simulink model "Simplified_UAV_Task3"  (R2024b)
settings: Solver=VariableStepAuto  StartTime=0  StopTime=3000  FixedStep=1e-4  RelTol=1e-5  AbsTol=1e-5
values from neighbouring files (symbols this model uses):
  adaptiveActivation = 1    [Simplified_UAV_Task3_main.m]    (also in newUAV_Task3_main.m)
  B_p = 1/UAV.m    [Simplified_UAV_Task3_main.m]    (also in newUAV_Task3_main.m)
  Gamma_a = 1*[1 1 1 1]'    [Simplified_UAV_Task3_main.m]    (also in newUAV_Task3_main.m = 2*[1 1 1 1]')
  gravityInAdaptiveController = 1    [Simplified_UAV_Task3_main.m]    (also in newUAV_Task3_main.m)
  L = 10    [Simplified_UAV_Task3_main.m]    (also in newUAV_Task3_main.m)
  lambda = 0.89    [Simplified_UAV_Task3_main.m]    (also in newUAV_Task3_main.m)
  lambda_0 = 1    [Simplified_UAV_Task3_main.m]    (also in newUAV_Task3_main.m)
  p_0 = [0; 0; 0]    [Simplified_UAV_Task3_main.m]    (also in newUAV_Task3_main.m)
  PO = 1    [Simplified_UAV_Task3_main.m]    (also in newUAV_Task3_main.m)
  scenario = 2    [Simplified_UAV_Task3_main.m]    (also in newUAV_Task3_main.m)
  theta_0 = [0.07;0.07;0.1]    [Simplified_UAV_Task3_main.m]    (also in newUAV_Task3_main.m)
  vb_0 = [0; 0; 0]    [Simplified_UAV_Task3_main.m]    (also in newUAV_Task3_main.m)
undefined symbols (not defined in the file or in its folder): ctrl, epsilon_PO, g, Gamma_a_scalar, par, projection_operator, targetParams, theta_M, UAV, v_0
libraries: matrix_library x12, slpidlib x12, spsRMSLib x1, uavutilslib x1
(part 1 of 3)
settings Model: Creator=justs  LastModifiedBy=giuseppe
settings SolverCC: ZeroCrossAlgorithm=Adaptive
settings DataIOCC: SaveFormat=StructureWithTime
settings OptimizationCC: BlockReduction=off  BufferReuse=off  ReuseModelBlockBuffer=off
settings DebuggingCC: AlgebraicLoopMsg=none
settings ModelReferenceCC: EnableRefExpFcnMdlSchedulingChecks=on
settings RTWCC: GPUComputeCapability=3.5

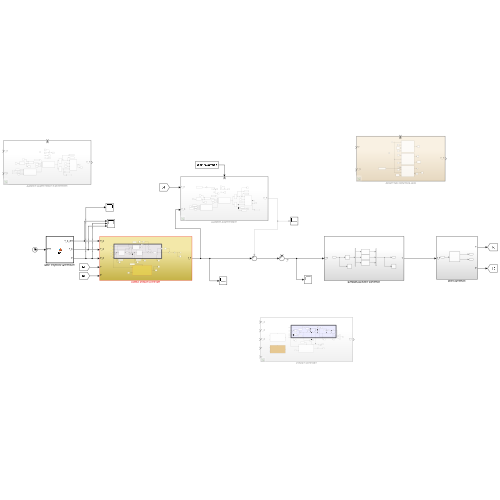
[thumbnail: Simulink's stored preview of the top-level diagram]
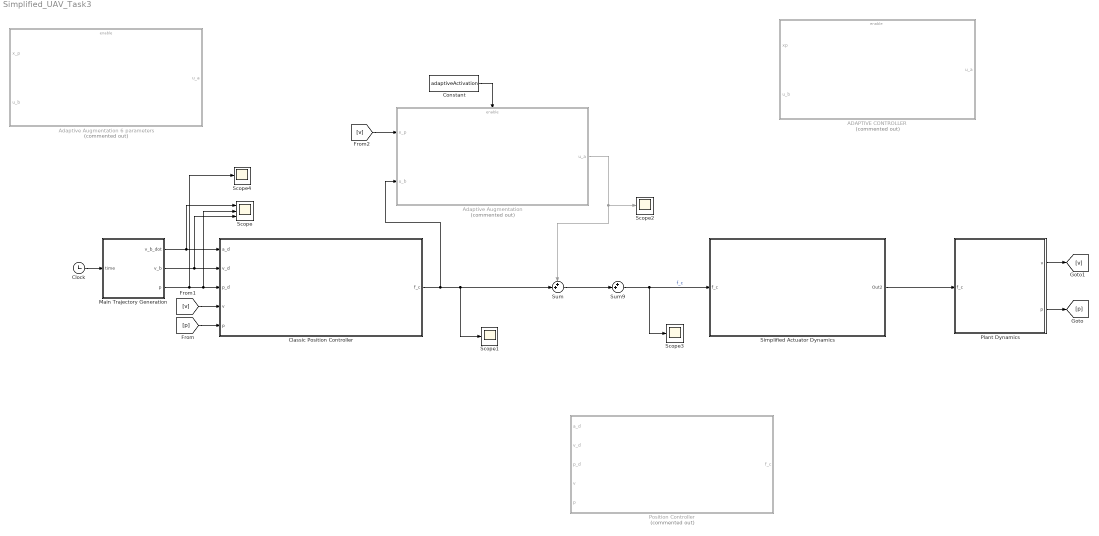
== system Simplified_UAV_Task3 ==
  ADAPTIVE CONTROLLER : Subsystem  Commented=on
  Adaptive Augmentation : Subsystem  Commented=on
  Adaptive Augmentation 6 parameters : Subsystem  Commented=on
  Classic Position Controller : Subsystem
  Clock : Clock
  Constant : Constant  Value=adaptiveActivation
  Main Trajectory Generation : MATLAB Function  TreatAsAtomicUnit=on
  Plant Dynamics : Subsystem
  Position Controller : Subsystem  Commented=on
  Scope : Scope  NumInputPorts=3
  Scope{1..4} (4 alike) : Scope
  Simplified Actuator Dynamics : Subsystem
  Sum : Sum  Inputs=++|
  Sum9 : Sum  Inputs=++|
  wires:
  Clock/1 -> Main Trajectory Generation/1(time)
  Simplified Actuator Dynamics/1(Out2) -> Plant Dynamics/1(f_c)
  Main Trajectory Generation/1(v_b_dot) -> Classic Position Controller/1(a_d), Scope/1
  Main Trajectory Generation/3(p) -> Scope4/1, Classic Position Controller/3(p_d), Scope/2
  Plant Dynamics/2(p) -> [p]
  [p] -> Classic Position Controller/5(p)
  Plant Dynamics/1(v) -> [v]
  [v] -> Classic Position Controller/4(v)
  Main Trajectory Generation/2(v_b) -> Classic Position Controller/2(v_d), Scope/3
  Classic Position Controller/1(f_c) -> Adaptive Augmentation/2(u_b), Scope1/1, Sum/2
  [v] -> Adaptive Augmentation/1(x_p)
  Adaptive Augmentation/1(u_a) -> Scope2/1, Sum/1
  Constant/1 -> Adaptive Augmentation/Enable
  Sum/1 -> Sum9/2
  Sum9/1 -> Scope3/1, Simplified Actuator Dynamics/1(f_c)  "f_c"

== system Simplified_UAV_Task3/ADAPTIVE CONTROLLER ==
  xp : Inport
  u_b : Inport  Port=2
  Enable : EnablePort
  Constant2 : Constant  Value=UAV.m*g*e3
  Scope : Scope
  Subsystem : Subsystem
  Subsystem1 : Subsystem
  Subsystem2 : Subsystem
  Sum : Sum  Inputs=|++
  u_a : Outport
  wires:
  Subsystem/1(xp_hat) -> [xp_hat]
  [thetap_hat] -> Subsystem1/4(thetap_hat)
  [thetap_hat] -> Subsystem/3(thetap_hat)
  xp/1 -> Subsystem1/3(xp), Subsystem2/2(xp), Subsystem/1(xp)
  [xp_hat] -> Subsystem2/3(xp_hat)
  [lambda] -> Subsystem/2(lambda)
  [u] -> Subsystem2/1(u)
  [u] -> Subsystem/4(u)
  Subsystem1/2(u) -> Scope/1, [u]
  [lambda] -> Subsystem1/2(lambda)
  Subsystem1/1(u_a) -> u_a/1
  Subsystem2/1(lambda) -> [lambda]
  Subsystem2/2(thetap_hat) -> [thetap_hat]
  Constant2/1 -> Sum/2
  u_b/1 -> Sum/1
  Sum/1 -> Subsystem1/1(u_b)

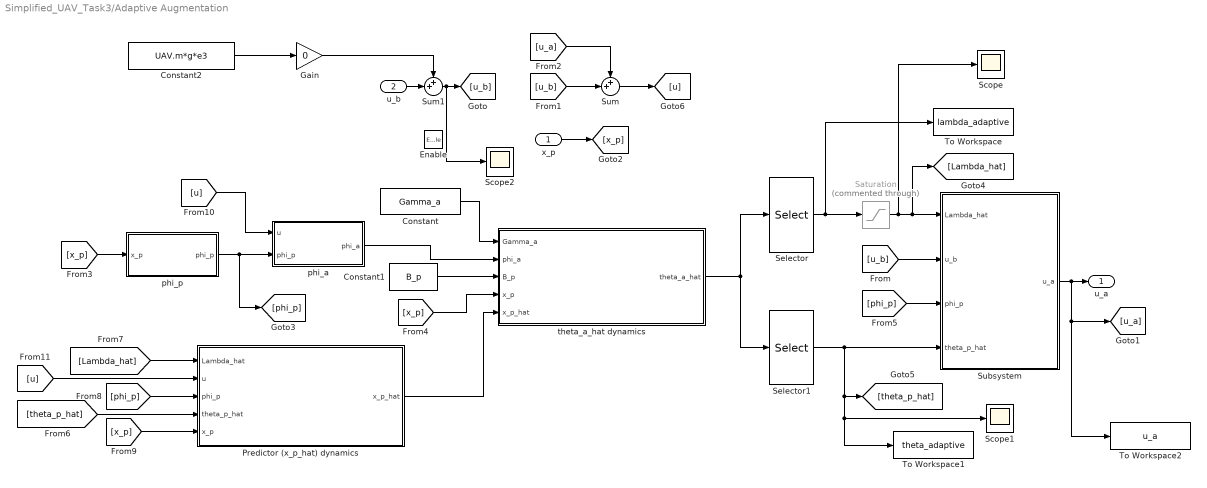
== system Simplified_UAV_Task3/Adaptive Augmentation ==
  x_p : Inport
  u_b : Inport  Port=2
  Enable : EnablePort
  Constant : Constant  Value=Gamma_a
  Constant1 : Constant  Value=B_p
  Constant2 : Constant  Value=UAV.m*g*e3
  Gain : Gain  Gain=0
  Predictor (x_p_hat) dynamics : Subsystem
  Saturation : Saturate  Commented=through  UpperLimit=1.5  LowerLimit=0.5
  Scope : Scope
  Scope1 : Scope
  Scope2 : Scope
  Selector : Selector  InputPortWidth=4  IndexOptions=Index vector (dialog)  Indices=[1]  OutputSizes=1
  Selector1 : Selector  InputPortWidth=4  IndexOptions=Index vector (dialog)  Indices=[2 3 4]  OutputSizes=1
  Subsystem : Subsystem
  Sum : Sum  Inputs=++|
  Sum1 : Sum  Inputs=++|
  To Workspace : ToWorkspace  VariableName=lambda_adaptive  SaveFormat=Timeseries  SampleTime=-1
  To Workspace1 : ToWorkspace  VariableName=theta_adaptive  SaveFormat=Timeseries  SampleTime=-1
  To Workspace2 : ToWorkspace  VariableName=u_a  SaveFormat=Timeseries  SampleTime=-1
  phi_a : Subsystem
  phi_p : Subsystem
  theta_a_hat dynamics : Subsystem
  u_a : Outport
  wires:
  Subsystem/1(u_a) -> To Workspace2/1, [u_a], u_a/1
  Selector1/1 -> Scope1/1, To Workspace1/1, [theta_p_hat], Subsystem/4(theta_p_hat)
  theta_a_hat dynamics/1(theta_a_hat) -> Selector/1, Selector1/1
  Constant/1 -> theta_a_hat dynamics/1(Gamma_a)
  phi_p/1(phi_p) -> phi_a/2(phi_p), [phi_p]
  [u_b] -> Sum/2
  phi_a/1(phi_a) -> theta_a_hat dynamics/2(phi_a)
  [x_p] -> phi_p/1(x_p)
  [x_p] -> theta_a_hat dynamics/4(x_p)
  Constant1/1 -> theta_a_hat dynamics/3(B_p)
  [phi_p] -> Subsystem/3(phi_p)
  Predictor (x_p_hat) dynamics/1(x_p_hat) -> theta_a_hat dynamics/5(x_p_hat)
  [theta_p_hat] -> Predictor (x_p_hat) dynamics/4(theta_p_hat)
  [Lambda_hat] -> Predictor (x_p_hat) dynamics/1(Lambda_hat)
  [phi_p] -> Predictor (x_p_hat) dynamics/3(phi_p)
  [x_p] -> Predictor (x_p_hat) dynamics/5(x_p)
  Sum/1 -> [u]
  [u] -> Predictor (x_p_hat) dynamics/2(u)
  Selector/1 -> To Workspace/1, Saturation/1
  x_p/1 -> [x_p]
  [u_a] -> Sum/1
  [u] -> phi_a/1(u)
  Saturation/1 -> Scope/1, [Lambda_hat], Subsystem/1(Lambda_hat)
  u_b/1 -> Sum1/2
  Sum1/1 -> Scope2/1, [u_b]
  Constant2/1 -> Gain/1
  Gain/1 -> Sum1/1
  [u_b] -> Subsystem/2(u_b)

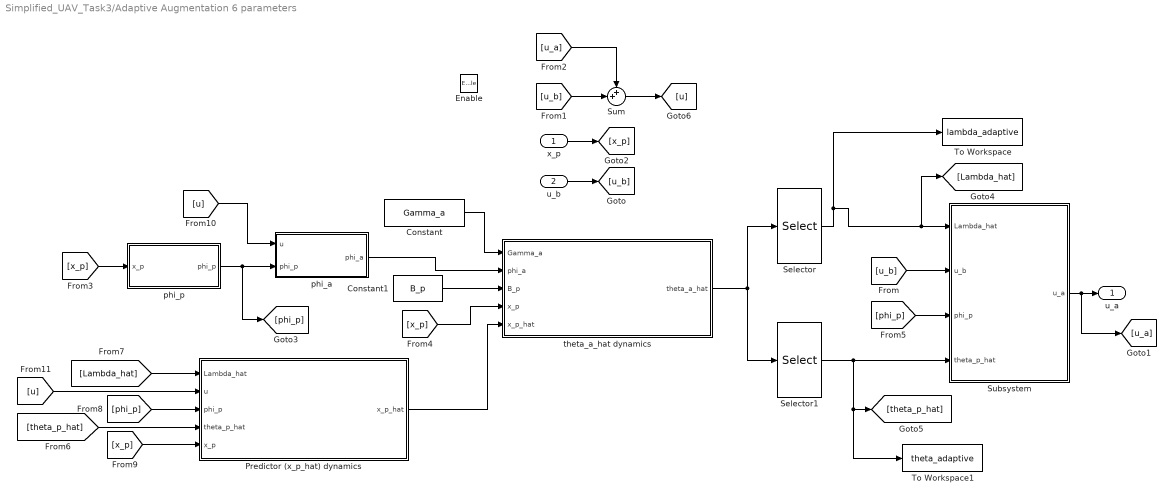
== system Simplified_UAV_Task3/Adaptive Augmentation 6 parameters ==
  x_p : Inport
  u_b : Inport  Port=2
  Enable : EnablePort
  Constant : Constant  Value=Gamma_a
  Constant1 : Constant  Value=B_p
  Predictor (x_p_hat) dynamics : Subsystem
  Selector : Selector  InputPortWidth=4  IndexOptions=Index vector (dialog)  Indices=[1]  OutputSizes=1
  Selector1 : Selector  InputPortWidth=4  IndexOptions=Index vector (dialog)  Indices=[2 3 4]  OutputSizes=1
  Subsystem : Subsystem
  Sum : Sum  Inputs=++|
  To Workspace : ToWorkspace  VariableName=lambda_adaptive  SaveFormat=Timeseries  SampleTime=-1
  To Workspace1 : ToWorkspace  VariableName=theta_adaptive  SaveFormat=Timeseries  SampleTime=-1
  phi_a : Subsystem
  phi_p : Subsystem
  theta_a_hat dynamics : Subsystem
  u_a : Outport
  wires:
  Subsystem/1(u_a) -> [u_a], u_a/1
  Selector1/1 -> To Workspace1/1, [theta_p_hat], Subsystem/4(theta_p_hat)
  theta_a_hat dynamics/1(theta_a_hat) -> Selector/1, Selector1/1
  Constant/1 -> theta_a_hat dynamics/1(Gamma_a)
  phi_p/1(phi_p) -> phi_a/2(phi_p), [phi_p]
  u_b/1 -> [u_b]
  [u_b] -> Subsystem/2(u_b)
  [u_b] -> Sum/2
  phi_a/1(phi_a) -> theta_a_hat dynamics/2(phi_a)
  [x_p] -> phi_p/1(x_p)
  [x_p] -> theta_a_hat dynamics/4(x_p)
  Constant1/1 -> theta_a_hat dynamics/3(B_p)
  [phi_p] -> Subsystem/3(phi_p)
  Predictor (x_p_hat) dynamics/1(x_p_hat) -> theta_a_hat dynamics/5(x_p_hat)
  [theta_p_hat] -> Predictor (x_p_hat) dynamics/4(theta_p_hat)
  [Lambda_hat] -> Predictor (x_p_hat) dynamics/1(Lambda_hat)
  [phi_p] -> Predictor (x_p_hat) dynamics/3(phi_p)
  [x_p] -> Predictor (x_p_hat) dynamics/5(x_p)
  Sum/1 -> [u]
  [u] -> Predictor (x_p_hat) dynamics/2(u)
  Selector/1 -> [Lambda_hat], Subsystem/1(Lambda_hat), To Workspace/1
  x_p/1 -> [x_p]
  [u_a] -> Sum/1
  [u] -> phi_a/1(u)

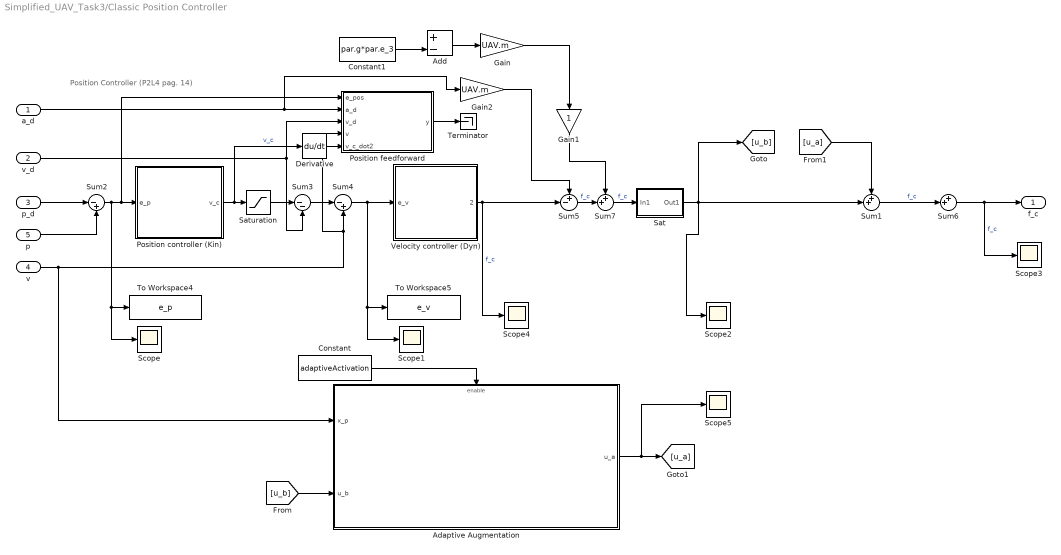
== system Simplified_UAV_Task3/Classic Position Controller ==
  note: Position Controller (P2L4 pag. 14)
  a_d : Inport
  v_d : Inport  Port=2
  p_d : Inport  Port=3
  v : Inport  Port=4
  p : Inport  Port=5
  Adaptive Augmentation : Subsystem
  Add : Sum  Inputs=+-
  Constant : Constant  Value=adaptiveActivation
  Constant1 : Constant  Value=par.g*par.e_3
  Derivative : Derivative
  Gain : Gain  Gain=UAV.m
  Gain1 : Gain
  Gain2 : Gain  Gain=UAV.m
  Position controller (Kin) : Subsystem
  Position feedforward : MATLAB Function  TreatAsAtomicUnit=on
  Sat : Subsystem
  Saturation : Saturate  UpperLimit=ctrl.vMax  LowerLimit=-ctrl.vMax
  Scope{,1..5} (6 alike) : Scope
  Sum1 : Sum  Inputs=++|
  Sum2 : Sum  Inputs=|-+
  Sum3 : Sum  Inputs=|--
  Sum4 : Sum  Inputs=|-+
  Sum5 : Sum  Inputs=+-|
  Sum6 : Sum  Inputs=++|
  Sum7 : Sum  Inputs=++|
  Terminator : Terminator
  To Workspace4 : ToWorkspace  VariableName=e_p  SaveFormat=Timeseries  SampleTime=-1
  To Workspace5 : ToWorkspace  VariableName=e_v  SaveFormat=Timeseries  SampleTime=-1
  Velocity controller (Dyn) : Subsystem
  f_c : Outport
  wires:
  p/1 -> Sum2/2
  a_d/1 -> Gain2/1, Position feedforward/2(a_d)
  Sum4/1 -> Scope1/1, To Workspace5/1, Velocity controller (Dyn)/1(e_v)
  v_d/1 -> Sum3/2, Position feedforward/3(v_d)
  p_d/1 -> Sum2/1
  Sum3/1 -> Sum4/1
  Sum2/1 -> Position feedforward/1(e_pos), Position controller (Kin)/1(e_p), Scope/1, To Workspace4/1
  Sum5/1 -> Sum7/2  "f_c"
  Position controller (Kin)/1(v_c) -> Derivative/1, Saturation/1  "v_c"
  Saturation/1 -> Sum3/1
  Velocity controller (Dyn)/1(2) -> Scope4/1, Sum5/2  "f_c"
  Derivative/1 -> Position feedforward/5(v_c_dot2)
  Position feedforward/1(y) -> Terminator/1
  Gain/1 -> Gain1/1
  Add/1 -> Gain/1
  Constant1/1 -> Add/2
  Sat/1(Out1) -> Scope2/1, [u_b], Sum1/2
  Gain1/1 -> Sum7/1
  Sum1/1 -> Sum6/2  "f_c"
  [u_b] -> Adaptive Augmentation/2(u_b)
  Adaptive Augmentation/1(u_a) -> Scope5/1, [u_a]
  [u_a] -> Sum1/1
  v/1 -> Adaptive Augmentation/1(x_p), Position feedforward/4(v), Sum4/2
  Constant/1 -> Adaptive Augmentation/Enable
  Sum6/1 -> Scope3/1, f_c/1  "f_c"
  Gain2/1 -> Sum5/1
  Sum7/1 -> Sat/1(In1)  "f_c"

== system Simplified_UAV_Task3/Plant Dynamics ==
  f_c : Inport
  Dynamics : Subsystem
  v : Outport
  p : Outport  Port=2
  wires:
  Dynamics/1(p) -> p/1
  Dynamics/2(v) -> v/1
  f_c/1 -> Dynamics/1(f_c)

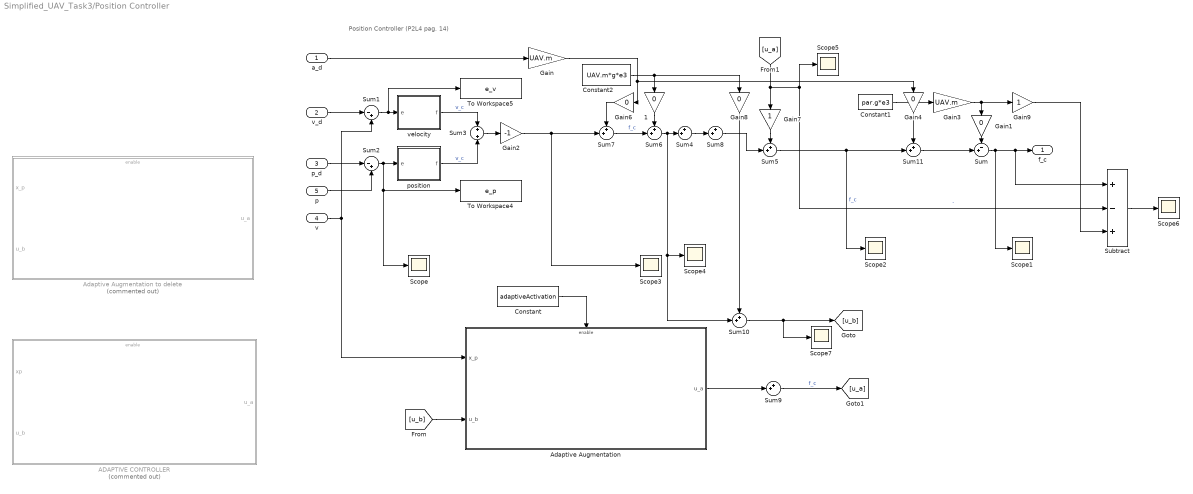
== system Simplified_UAV_Task3/Position Controller ==
  note: Position Controller (P2L4 pag. 14)
  a_d : Inport
  v_d : Inport  Port=2
  p_d : Inport  Port=3
  v : Inport  Port=4
  p : Inport  Port=5
  1 : Gain  Gain=0
  ADAPTIVE CONTROLLER : Subsystem  Commented=on
  Adaptive Augmentation : Subsystem
  Adaptive Augmentation to delete : Subsystem  Commented=on
  Constant : Constant  Value=adaptiveActivation
  "Constant1 " : Constant  Value=par.g*e3
  Constant2 : Constant  Value=UAV.m*g*e3
  Gain : Gain  Gain=UAV.m
  Gain{1,4,6,8} (4 alike) : Gain  Gain=0
  Gain2 : Gain  Gain=-1
  Gain3 : Gain  Gain=UAV.m
  Gain7 : Gain
  Gain9 : Gain
  Scope{,1..7} (8 alike) : Scope
  Subtract : Sum  Inputs=+-+
  Sum : Sum  Inputs=-+|
  Sum1 : Sum  Inputs=|-+
  Sum{4..11} (8 alike) : Sum  Inputs=++|
  Sum2 : Sum  Inputs=|-+
  Sum3 : Sum  Inputs=+|+
  To Workspace4 : ToWorkspace  VariableName=e_p  SaveFormat=Timeseries  SampleTime=-1
  To Workspace5 : ToWorkspace  VariableName=e_v  SaveFormat=Timeseries  SampleTime=-1
  position : Subsystem
  velocity : Subsystem
  f_c : Outport
  wires:
  p/1 -> Sum2/2
  v/1 -> Adaptive Augmentation/1(x_p), Sum1/2
  p_d/1 -> Sum2/1
  Sum2/1 -> position/1(e), Scope/1, To Workspace4/1
  Sum5/1 -> Sum11/2, Scope2/1  "f_c"
  Constant/1 -> Adaptive Augmentation/Enable
  [u_b] -> Adaptive Augmentation/2(u_b)
  [u_a] -> Subtract/2, Scope5/1, Gain7/1  "-"
  Gain/1 -> Gain6/1, Gain4/1
  a_d/1 -> Gain/1
  "Constant1 "/1 -> Gain3/1
  Sum/1 -> Scope1/1, Subtract/1, f_c/1
  v_d/1 -> Sum1/1
  Sum1/1 -> velocity/1(e), To Workspace5/1
  velocity/1(f) -> Sum3/1  "v_c"
  position/1(f) -> Sum3/2  "v_c"
  Sum3/1 -> Gain2/1
  Gain3/1 -> Gain9/1, Gain1/1
  Gain1/1 -> Sum/1
  Gain4/1 -> Sum11/1
  Gain2/1 -> Scope3/1, Sum7/2
  Constant2/1 -> Gain8/1, 1/1
  Sum7/1 -> Sum6/2  "f_c"
  Gain6/1 -> Sum7/1
  Gain7/1 -> Sum5/1
  Gain8/1 -> Sum10/1
  Sum4/1 -> Sum8/2
  Sum6/1 -> Sum10/2, Scope4/1, Sum4/2
  Subtract/1 -> Scope6/1
  Gain9/1 -> Subtract/3
  Adaptive Augmentation/1(u_a) -> Sum9/2
  Sum9/1 -> [u_a]  "f_c"
  Sum8/1 -> Sum5/2
  Sum10/1 -> Scope7/1, [u_b]
  1/1 -> Sum6/1
  Sum11/1 -> Sum/2

== system Simplified_UAV_Task3/Simplified Actuator Dynamics ==
  f_c : Inport
  Demux : Demux  Outputs=3
  Mux : Mux  Inputs=3
  Saturation : Saturate  UpperLimit=6  LowerLimit=-6
  Scope1 : Scope
  Scope2 : Scope
  Transfer Fcn : TransferFcn  Denominator=[1/70 1]
  Transfer Fcn1 : TransferFcn  Denominator=[1/10 1]
  Transfer Fcn2 : TransferFcn  Denominator=[1/10 1]
  Out2 : Outport
  wires:
  f_c/1 -> Saturation/1, Scope2/1
  Mux/1 -> Scope1/1, Out2/1
  Demux/1 -> Transfer Fcn2/1
  Demux/2 -> Transfer Fcn1/1
  Transfer Fcn/1 -> Mux/3
  Demux/3 -> Transfer Fcn/1
  Transfer Fcn1/1 -> Mux/2
  Transfer Fcn2/1 -> Mux/1
  Saturation/1 -> Demux/1

== system Simplified_UAV_Task3/ADAPTIVE CONTROLLER/Subsystem ==
  xp : Inport
  lambda : Inport  Port=2
  thetap_hat : Inport  Port=3
  u : Inport  Port=4
  Constant : Constant  Value=[0 0 g]'
  Create Diagonal Matrix : matrix_library/Create Diagonal Matrix
  Gain : Gain  Gain=B_p
  Gain1 : Gain  Gain=L
  Gain2 : Gain  Gain=-1
  Integrator : Integrator
  MATLAB Function1 : MATLAB Function  Commented=through  TreatAsAtomicUnit=on
  Matrix Multiply : Product  Multiplication=Matrix(*)
  Matrix Multiply1 : Product
  Scope : Scope
  Sum : Sum
  Sum1 : Sum  Inputs=+++
  Sum2 : Sum  Inputs=+-
  xp_hat : Outport
  wires:
  xp/1 -> Sum2/1, Create Diagonal Matrix/1
  thetap_hat/1 -> Matrix Multiply/2
  u/1 -> Matrix Multiply1/2
  MATLAB Function1/1(Lambda_hat) -> Matrix Multiply1/1
  lambda/1 -> MATLAB Function1/1(lambda)
  Sum/1 -> Gain/1
  Matrix Multiply1/1 -> Sum/1
  Matrix Multiply/1 -> Sum/2
  Gain/1 -> Sum1/2
  Constant/1 -> Sum1/1
  Integrator/1 -> xp_hat/1, Sum2/2
  Sum2/1 -> Scope/1, Gain1/1
  Gain1/1 -> Sum1/3
  Sum1/1 -> Integrator/1
  Create Diagonal Matrix/1 -> Gain2/1
  Gain2/1 -> Matrix Multiply/1

== system Simplified_UAV_Task3/ADAPTIVE CONTROLLER/Subsystem1 ==
  u_b : Inport
  lambda : Inport  Port=2
  xp : Inport  Port=3
  thetap_hat : Inport  Port=4
  Constant : Constant
  Create Diagonal Matrix : matrix_library/Create Diagonal Matrix
  Gain2 : Gain  Gain=-1
  MATLAB Function1 : MATLAB Function  TreatAsAtomicUnit=on
  Matrix Multiply : Product
  Matrix Multiply1 : Product  Multiplication=Matrix(*)
  Matrix Multiply2 : Product
  Sum : Sum  Inputs=+-
  Sum1 : Sum  Inputs=+-
  Sum2 : Sum
  u_a : Outport
  u : Outport  Port=2
  wires:
  lambda/1 -> MATLAB Function1/1(lambda)
  MATLAB Function1/1(Lambda_hat_inv) -> Matrix Multiply2/1, Sum/1
  Constant/1 -> Sum/2
  Sum/1 -> Matrix Multiply/1
  u_b/1 -> Sum2/2, Matrix Multiply/2
  Matrix Multiply/1 -> Sum1/1
  xp/1 -> Create Diagonal Matrix/1
  thetap_hat/1 -> Matrix Multiply1/2
  Sum1/1 -> Sum2/1, u_a/1
  Sum2/1 -> u/1
  Create Diagonal Matrix/1 -> Gain2/1
  Gain2/1 -> Matrix Multiply1/1
  Matrix Multiply1/1 -> Matrix Multiply2/2
  Matrix Multiply2/1 -> Sum1/2

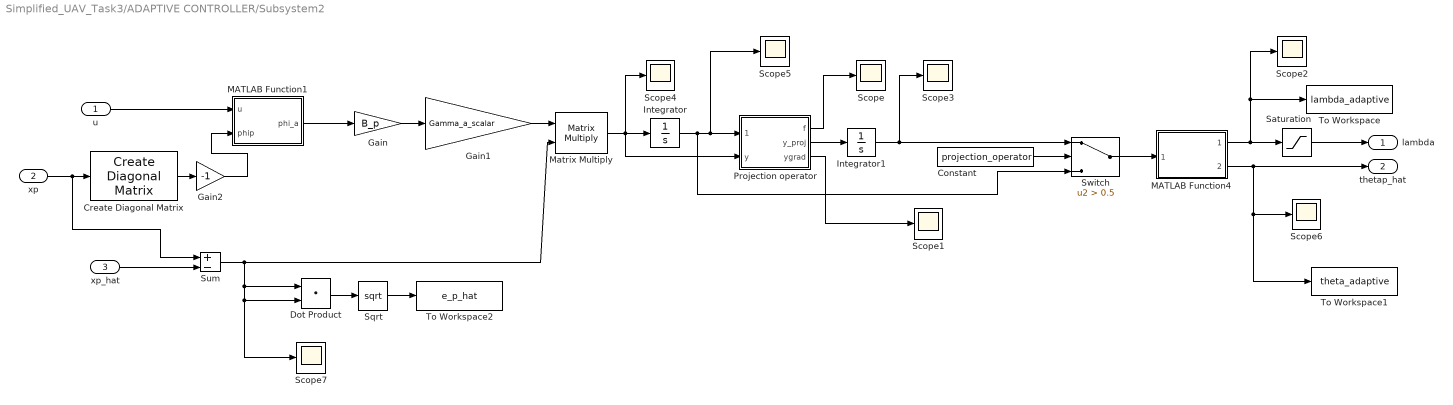
== system Simplified_UAV_Task3/ADAPTIVE CONTROLLER/Subsystem2 ==
  u : Inport
  xp : Inport  Port=2
  xp_hat : Inport  Port=3
  Constant : Constant  Value=projection_operator
  Create Diagonal Matrix : matrix_library/Create Diagonal Matrix
  Dot Product : DotProduct  OutDataTypeStr=Inherit: Inherit via internal rule
  Gain : Gain  Gain=B_p
  Gain1 : Gain  Gain=Gamma_a_scalar
  Gain2 : Gain  Gain=-1
  Integrator : Integrator  InitialCondition=[lambda_0; theta_0]
  Integrator1 : Integrator  InitialCondition=[1 0.07 0.07 0.1]'
  MATLAB Function1 : MATLAB Function  TreatAsAtomicUnit=on
  MATLAB Function4 : MATLAB Function  TreatAsAtomicUnit=on
  Matrix Multiply : Product  Multiplication=Matrix(*)
  Projection operator : MATLAB Function  TreatAsAtomicUnit=on
  Saturation : Saturate  UpperLimit=1.5  LowerLimit=0.5
  Scope{,1..7} (8 alike) : Scope
  Sqrt : Sqrt
  Sum : Sum  Inputs=+-
  Switch : Switch  Criteria=u2 > Threshold  Threshold=0.5  SaturateOnIntegerOverflow=off  InputSameDT=off
  To Workspace : ToWorkspace  VariableName=lambda_adaptive  SaveFormat=Timeseries  SampleTime=-1
  To Workspace1 : ToWorkspace  VariableName=theta_adaptive  SaveFormat=Timeseries  SampleTime=-1
  To Workspace2 : ToWorkspace  VariableName=e_p_hat  SaveFormat=Timeseries  SampleTime=-1
  lambda : Outport
  thetap_hat : Outport  Port=2
  wires:
  u/1 -> MATLAB Function1/1(u)
  xp_hat/1 -> Sum/2
  MATLAB Function1/1(phi_a) -> Gain/1
  Gain/1 -> Gain1/1
  Gain1/1 -> Matrix Multiply/1
  Matrix Multiply/1 -> Projection operator/2(y), Scope4/1, Integrator/1
  MATLAB Function4/1(lambda) -> To Workspace/1, Scope2/1, Saturation/1
  Integrator/1 -> Switch/3, Scope5/1, Projection operator/1(theta_a_hat)
  Projection operator/3(ygrad) -> Scope1/1
  Projection operator/1(f) -> Scope/1
  MATLAB Function4/2(thetap_hat) -> To Workspace1/1, Scope6/1, thetap_hat/1
  Integrator1/1 -> Switch/1, Scope3/1
  Projection operator/2(y_proj) -> Integrator1/1
  xp/1 -> Create Diagonal Matrix/1, Sum/1
  Switch/1 -> MATLAB Function4/1(theta_a)
  Constant/1 -> Switch/2
  Create Diagonal Matrix/1 -> Gain2/1
  Gain2/1 -> MATLAB Function1/2(phip)
  Sqrt/1 -> To Workspace2/1
  Sum/1 -> Scope7/1, Dot Product/2, Dot Product/1, Matrix Multiply/2
  Dot Product/1 -> Sqrt/1
  Saturation/1 -> lambda/1

== system Simplified_UAV_Task3/Adaptive Augmentation/Predictor (x_p_hat) dynamics ==
  Lambda_hat : Inport
  u : Inport  Port=2
  phi_p : Inport  Port=3
  theta_p_hat : Inport  Port=4
  x_p : Inport  Port=5
  Add : Sum
  Constant : Constant  Value=g*e3
  Gain : Gain  Gain=B_p  Multiplication=Matrix(K*u)
  Gain1 : Gain  Gain=L
  Gain2 : Gain  Gain=gravityInAdaptiveController
  Integrator : Integrator  InitialCondition=v_0
  Matrix Multiply : Product
  Matrix Multiply1 : Product  Multiplication=Matrix(*)
  Reshape : Reshape  OutputDimensionality=Column vector (2-D)
  Reshape1 : Reshape  OutputDimensionality=Column vector (2-D)
  Reshape2 : Reshape  OutputDimensionality=Column vector (2-D)
  Scope : Scope
  Sum : Sum  Inputs=+++
  Sum1 : Sum  Inputs=-+|
  Transpose : Math  Operator=transpose
  x_p_hat : Outport
  wires:
  Lambda_hat/1 -> Matrix Multiply/1
  Matrix Multiply/1 -> Add/1
  phi_p/1 -> Transpose/1
  theta_p_hat/1 -> Matrix Multiply1/2
  Matrix Multiply1/1 -> Add/2
  Add/1 -> Gain/1
  Gain/1 -> Reshape1/1
  Gain1/1 -> Reshape/1
  x_p/1 -> Sum1/2
  Sum1/1 -> Gain1/1
  Integrator/1 -> Scope/1, Sum1/1, x_p_hat/1
  Sum/1 -> Integrator/1
  Reshape/1 -> Sum/1
  Reshape1/1 -> Sum/2
  Reshape2/1 -> Sum/3
  Constant/1 -> Gain2/1
  Transpose/1 -> Matrix Multiply1/1
  Gain2/1 -> Reshape2/1
  u/1 -> Matrix Multiply/2

== system Simplified_UAV_Task3/Adaptive Augmentation/Subsystem ==
  Lambda_hat : Inport
  u_b : Inport  Port=2
  phi_p : Inport  Port=3
  theta_p_hat : Inport  Port=4
  Constant : Constant  Value=eye(3,3)
  Gain : Gain  Commented=through  Gain=-1
  Gain1 : Gain
  Inverse : MATLAB Function  TreatAsAtomicUnit=on
  Product : Product  Multiplication=Matrix(*)
  Product1 : Product  Inputs=3  Multiplication=Matrix(*)
  Subtract : Sum  Inputs=-+
  Subtract1 : Sum  Inputs=+-
  Transpose : Math  Operator=transpose
  u_a : Outport
  wires:
  Lambda_hat/1 -> Inverse/1(u)
  Inverse/1(y) -> Product1/1, Subtract/2
  Constant/1 -> Subtract/1
  Subtract/1 -> Product/1
  u_b/1 -> Product/2
  Product/1 -> Gain1/1
  Subtract1/1 -> u_a/1
  phi_p/1 -> Transpose/1
  Transpose/1 -> Gain/1
  theta_p_hat/1 -> Product1/3
  Product1/1 -> Subtract1/2
  Gain/1 -> Product1/2
  Gain1/1 -> Subtract1/1

== system Simplified_UAV_Task3/Adaptive Augmentation/phi_a ==
  u : Inport
  phi_p : Inport  Port=2
  Matrix Concatenate : Concatenate  Mode=Multidimensional array
  Scope : Scope
  Transpose : Math  Operator=transpose
  phi_a : Outport
  wires:
  Matrix Concatenate/1 -> Scope/1, phi_a/1
  u/1 -> Transpose/1
  phi_p/1 -> Matrix Concatenate/2
  Transpose/1 -> Matrix Concatenate/1

== system Simplified_UAV_Task3/Adaptive Augmentation/phi_p ==
  x_p : Inport
  Create Diagonal Matrix : matrix_library/Create Diagonal Matrix
  Gain : Gain  Gain=-1
  phi_p : Outport
  wires:
  x_p/1 -> Gain/1
  Gain/1 -> Create Diagonal Matrix/1
  Create Diagonal Matrix/1 -> phi_p/1

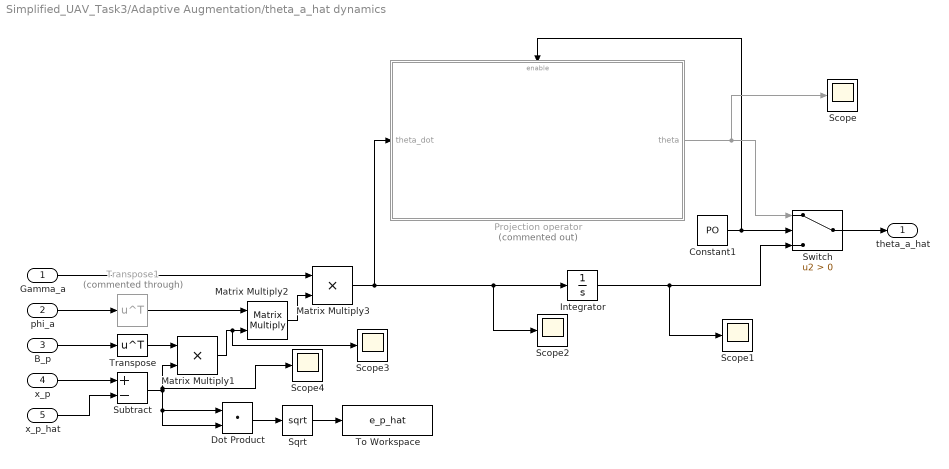
== system Simplified_UAV_Task3/Adaptive Augmentation/theta_a_hat dynamics ==
  Gamma_a : Inport
  phi_a : Inport  Port=2
  B_p : Inport  Port=3
  x_p : Inport  Port=4
  x_p_hat : Inport  Port=5
  Constant1 : Constant  Value=PO
  Dot Product : DotProduct  OutDataTypeStr=Inherit: Inherit via internal rule
  Integrator : Integrator  InitialCondition=[lambda_0; theta_0]
  Matrix Multiply1 : Product
  Matrix Multiply2 : Product  Multiplication=Matrix(*)
  Matrix Multiply3 : Product
  Projection operator : Subsystem  Commented=on
  Scope{,1..4} (5 alike) : Scope
  Sqrt : Sqrt
  Subtract : Sum  Inputs=+-
  Switch : Switch  Criteria=u2 > Threshold  SaturateOnIntegerOverflow=off  InputSameDT=off
  To Workspace : ToWorkspace  VariableName=e_p_hat  SaveFormat=Timeseries  SampleTime=-1
  Transpose : Math  Operator=transpose
  Transpose1 : Math  Commented=through  Operator=transpose
  theta_a_hat : Outport
  wires:
  x_p_hat/1 -> Subtract/2
  B_p/1 -> Transpose/1
  Subtract/1 -> Matrix Multiply1/2, Scope4/1, Dot Product/2, Dot Product/1
  Transpose/1 -> Matrix Multiply1/1
  phi_a/1 -> Transpose1/1
  Matrix Multiply1/1 -> Scope3/1, Matrix Multiply2/2
  Gamma_a/1 -> Matrix Multiply3/1
  Matrix Multiply2/1 -> Matrix Multiply3/2
  Matrix Multiply3/1 -> Projection operator/1(theta_dot), Scope2/1, Integrator/1
  x_p/1 -> Subtract/1
  Constant1/1 -> Switch/2, Projection operator/Enable
  Integrator/1 -> Scope1/1, Switch/3
  Switch/1 -> theta_a_hat/1
  Projection operator/1(theta) -> Scope/1, Switch/1
  Dot Product/1 -> Sqrt/1
  Sqrt/1 -> To Workspace/1
  Transpose1/1 -> Matrix Multiply2/1

== system Simplified_UAV_Task3/Adaptive Augmentation 6 parameters/Predictor (x_p_hat) dynamics ==
  Lambda_hat : Inport
  u : Inport  Port=2
  phi_p : Inport  Port=3
  theta_p_hat : Inport  Port=4
  x_p : Inport  Port=5
  Add : Sum
  Constant : Constant  Value=g*e3
  Gain : Gain  Gain=B_p  Multiplication=Matrix(K*u)
  Gain1 : Gain  Gain=L
  Integrator : Integrator  InitialCondition=v_0
  Matrix Multiply : Product  Multiplication=Matrix(*)
  Matrix Multiply1 : Product  Multiplication=Matrix(*)
  Reshape : Reshape  OutputDimensionality=Column vector (2-D)
  Reshape1 : Reshape  OutputDimensionality=Column vector (2-D)
  Reshape2 : Reshape  OutputDimensionality=Column vector (2-D)
  Sum : Sum  Inputs=+++
  Sum1 : Sum  Inputs=-+|
  Transpose : Math  Operator=transpose
  x_p_hat : Outport
  wires:
  Lambda_hat/1 -> Matrix Multiply/1
  u/1 -> Matrix Multiply/2
  Matrix Multiply/1 -> Add/1
  phi_p/1 -> Transpose/1
  theta_p_hat/1 -> Matrix Multiply1/2
  Matrix Multiply1/1 -> Add/2
  Transpose/1 -> Matrix Multiply1/1
  Add/1 -> Gain/1
  Gain/1 -> Reshape1/1
  Constant/1 -> Reshape2/1
  Gain1/1 -> Reshape/1
  x_p/1 -> Sum1/2
  Sum1/1 -> Gain1/1
  Integrator/1 -> Sum1/1, x_p_hat/1
  Sum/1 -> Integrator/1
  Reshape/1 -> Sum/1
  Reshape1/1 -> Sum/2
  Reshape2/1 -> Sum/3

== system Simplified_UAV_Task3/Adaptive Augmentation 6 parameters/Subsystem ==
  Lambda_hat : Inport
  u_b : Inport  Port=2
  phi_p : Inport  Port=3
  theta_p_hat : Inport  Port=4
  Constant : Constant  Value=eye(3,3)
  Inverse : MATLAB Function  TreatAsAtomicUnit=on
  Product : Product  Multiplication=Matrix(*)
  Product1 : Product  Multiplication=Matrix(*)
  Product2 : Product  Multiplication=Matrix(*)
  Subtract : Sum  Inputs=-+
  Subtract1 : Sum  Inputs=+-
  Transpose : Math  Operator=transpose
  u_a : Outport
  wires:
  Lambda_hat/1 -> Inverse/1(u)
  Inverse/1(y) -> Product1/1, Subtract/2
  Constant/1 -> Subtract/1
  Subtract/1 -> Product/1
  u_b/1 -> Product/2
  Product/1 -> Subtract1/1
  Subtract1/1 -> u_a/1
  phi_p/1 -> Transpose/1
  Transpose/1 -> Product2/1
  theta_p_hat/1 -> Product2/2
  Product2/1 -> Product1/2
  Product1/1 -> Subtract1/2

== system Simplified_UAV_Task3/Adaptive Augmentation 6 parameters/phi_a ==
  u : Inport
  phi_p : Inport  Port=2
  Create Diagonal Matrix : matrix_library/Create Diagonal Matrix
  Matrix Concatenate : Concatenate  Mode=Multidimensional array
  phi_a : Outport
  wires:
  phi_p/1 -> Matrix Concatenate/2
  u/1 -> Create Diagonal Matrix/1
  Matrix Concatenate/1 -> phi_a/1
  Create Diagonal Matrix/1 -> Matrix Concatenate/1

== system Simplified_UAV_Task3/Adaptive Augmentation 6 parameters/phi_p ==
  x_p : Inport
  Create Diagonal Matrix : matrix_library/Create Diagonal Matrix
  Gain : Gain  Gain=-1
  phi_p : Outport
  wires:
  x_p/1 -> Gain/1
  Gain/1 -> Create Diagonal Matrix/1
  Create Diagonal Matrix/1 -> phi_p/1

== system Simplified_UAV_Task3/Adaptive Augmentation 6 parameters/theta_a_hat dynamics ==
  Gamma_a : Inport
  phi_a : Inport  Port=2
  B_p : Inport  Port=3
  x_p : Inport  Port=4
  x_p_hat : Inport  Port=5
  Constant1 : Constant  Value=PO
  Integrator : Integrator  InitialCondition=[lambda_0; theta_0]
  Matrix Multiply1 : Product
  Matrix Multiply2 : Product  Multiplication=Matrix(*)
  Matrix Multiply3 : Product
  Projection operator : Subsystem  Commented=on
  Scope : Scope
  Subtract : Sum  Inputs=+-
  Switch : Switch  Criteria=u2 > Threshold  SaturateOnIntegerOverflow=off  InputSameDT=off
  Transpose : Math  Operator=transpose
  theta_a_hat : Outport
  wires:
  x_p_hat/1 -> Subtract/2
  B_p/1 -> Transpose/1
  Subtract/1 -> Matrix Multiply1/2
  Transpose/1 -> Matrix Multiply1/1
  phi_a/1 -> Matrix Multiply2/1
  Matrix Multiply1/1 -> Matrix Multiply2/2
  Gamma_a/1 -> Matrix Multiply3/1
  Matrix Multiply2/1 -> Matrix Multiply3/2
  Matrix Multiply3/1 -> Projection operator/1(theta_dot), Integrator/1
  x_p/1 -> Subtract/1
  Constant1/1 -> Switch/2, Projection operator/Enable
  Integrator/1 -> Switch/3
  Switch/1 -> theta_a_hat/1
  Projection operator/1(theta) -> Scope/1, Switch/1

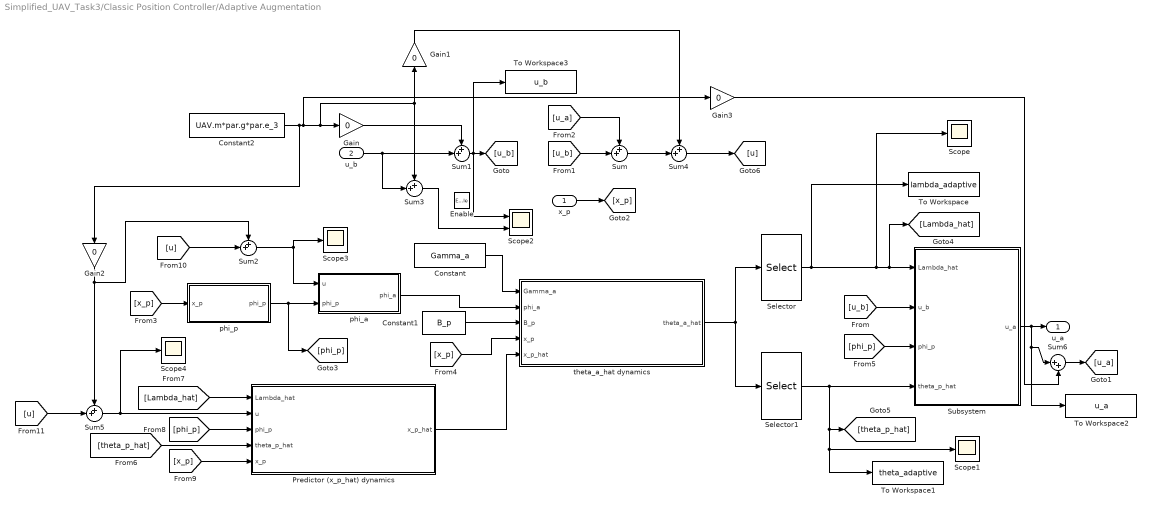
== system Simplified_UAV_Task3/Classic Position Controller/Adaptive Augmentation ==
  x_p : Inport
  u_b : Inport  Port=2
  Enable : EnablePort
  Constant : Constant  Value=Gamma_a
  Constant1 : Constant  Value=B_p
  Constant2 : Constant  Value=UAV.m*par.g*par.e_3
  Gain{,1..3} (4 alike) : Gain  Gain=0
  Predictor (x_p_hat) dynamics : Subsystem
  Scope{,1,3..4} (4 alike) : Scope
  Scope2 : Scope  NumInputPorts=2
  Selector : Selector  InputPortWidth=4  IndexOptions=Index vector (dialog)  Indices=[1]  OutputSizes=1
  Selector1 : Selector  InputPortWidth=4  IndexOptions=Index vector (dialog)  Indices=[2 3 4]  OutputSizes=1
  Subsystem : Subsystem
  Sum{,1..5} (6 alike) : Sum  Inputs=++|
  Sum6 : Sum  Inputs=|++
  To Workspace : ToWorkspace  VariableName=lambda_adaptive  SaveFormat=Timeseries  SampleTime=-1
  To Workspace1 : ToWorkspace  VariableName=theta_adaptive  SaveFormat=Timeseries  SampleTime=-1
  To Workspace2 : ToWorkspace  VariableName=u_a  SaveFormat=Timeseries  SampleTime=-1
  To Workspace3 : ToWorkspace  VariableName=u_b  SaveFormat=Timeseries  SampleTime=-1
  phi_a : Subsystem
  phi_p : Subsystem
  theta_a_hat dynamics : Subsystem
  u_a : Outport
  wires:
  Selector1/1 -> Scope1/1, To Workspace1/1, [theta_p_hat], Subsystem/4(theta_p_hat)
  theta_a_hat dynamics/1(theta_a_hat) -> Selector/1, Selector1/1
  Constant/1 -> theta_a_hat dynamics/1(Gamma_a)
  phi_p/1(phi_p) -> phi_a/2(phi_p), [phi_p]
  [u_b] -> Sum/2
  phi_a/1(phi_a) -> theta_a_hat dynamics/2(phi_a)
  [x_p] -> phi_p/1(x_p)
  [x_p] -> theta_a_hat dynamics/4(x_p)
  Constant1/1 -> theta_a_hat dynamics/3(B_p)
  [phi_p] -> Subsystem/3(phi_p)
  Predictor (x_p_hat) dynamics/1(x_p_hat) -> theta_a_hat dynamics/5(x_p_hat)
  [theta_p_hat] -> Predictor (x_p_hat) dynamics/4(theta_p_hat)
  [Lambda_hat] -> Predictor (x_p_hat) dynamics/1(Lambda_hat)
  [phi_p] -> Predictor (x_p_hat) dynamics/3(phi_p)
  [x_p] -> Predictor (x_p_hat) dynamics/5(x_p)
  x_p/1 -> [x_p]
  [u_a] -> Sum/1
  Selector/1 -> Scope/1, [Lambda_hat], Subsystem/1(Lambda_hat), To Workspace/1
  u_b/1 -> Sum3/2, Sum1/2
  Sum1/1 -> Scope2/1, To Workspace3/1, [u_b]
  [u_b] -> Subsystem/2(u_b)
  Subsystem/1(u_a) -> Sum6/1, To Workspace2/1, u_a/1
  Sum2/1 -> phi_a/1(u), Scope3/1
  [u] -> Sum2/2
  Gain/1 -> Sum1/1
  Sum3/1 -> Scope2/2
  Sum/1 -> Sum4/2
  Sum4/1 -> [u]
  Constant2/1 -> Gain2/1, Gain3/1, Gain1/1, Sum3/1, Gain/1
  Gain1/1 -> Sum4/1
  [u] -> Sum5/2
  Sum5/1 -> Scope4/1, Predictor (x_p_hat) dynamics/2(u)
  Gain2/1 -> Sum2/1, Sum5/1
  Sum6/1 -> [u_a]
  Gain3/1 -> Sum6/2

== system Simplified_UAV_Task3/Classic Position Controller/Position controller (Kin) ==
  e_p : Inport
  Constant : Constant  Value=scenario
  Demux : Demux  Outputs=3
  If : If  IfExpression=u1 == 2
  Mux : Mux  Inputs=3
  PID Controller x : slpidlib/PID Controller  Controller=P  Form=Parallel  TimeDomain=Continuous-time  UseExternalTs=off  SampleTime=-1  IntegratorMethod=Forward Euler  FilterMethod=Forward Euler  ControllerParametersSource=internal  P=ctrl.Kpos(1,1)  I=ctrl.Kipos(1,1)  UseKiTs=off  D=0  UseExternalDerivativeSource=off  N=100  UseFilter=on  TunerSelectOption=Transfer Function Based (PID Tuner App)  InitialConditionSource=internal  InitialConditionForIntegrator=0  InitialConditionForFilter=0  DifferentiatorICPrevScaledInput=0  ExternalReset=none  TrackingMode=off  Kt=1  LimitOutput=off  SatLimitsSource=internal  UpperSaturationLimit=inf  LowerSaturationLimit=-inf  LinearizeAsGain=on  AntiWindupMode=none  Kb=1  LimitIntegrator=off  UpperIntegratorSaturationLimit=inf  LowerIntegratorSaturationLimit=-inf  POutMin=[]  POutMax=[]  IOutMin=[]  IOutMax=[]  DOutMin=[]  DOutMax=[]  NOutMin=[]  NOutMax=[]  SumOutMin=[]  SumOutMax=[]  SaturationOutMin=[]  SaturationOutMax=[]  PParamMin=[]  PParamMax=[]  IParamMin=[]  IParamMax=[]  DParamMin=[]  DParamMax=[]  NParamMin=[]  NParamMax=[]  KbParamMin=[]  KbParamMax=[]  KtParamMin=[]  KtParamMax=[]  KbOutMin=[]  KbOutMax=[]  KtOutMin=[]  KtOutMax=[]  IntegratorOutMin=[]  IntegratorOutMax=[]  FilterOutMin=[]  FilterOutMax=[]  SumI1OutMin=[]  SumI1OutMax=[]  SumI2OutMin=[]  SumI2OutMax=[]  SumI3OutMin=[]  SumI3OutMax=[]  SumI4OutMin=[]  SumI4OutMax=[]  SumDOutMin=[]  SumDOutMax=[]  DifferentiatorOutMin=[]  DifferentiatorOutMax=[]  FilterDiffOutCoefMin=[]  FilterDiffOutCoefMax=[]  ReciprocalOutMin=[]  ReciprocalOutMax=[]  SumDenOutMin=[]  SumDenOutMax=[]  SumNumOutMin=[]  SumNumOutMax=[]  DivideOutMin=[]  DivideOutMax=[]  UdiffTsProdOutMin=[]  UdiffTsProdOutMax=[]  NTsProdOutMin=[]  NTsProdOutMax=[]  UintegralTsProdOutMin=[]  UintegralTsProdOutMax=[]  UngainTsProdOutMin=[]  UngainTsProdOutMax=[]  ClampingZeroOutDataTypeStr=Inherit: Inherit via back propagation  ClampingZeroOutMin=[]  ClampingZeroOutMax=[]  FilterDenConstantOutDataTypeStr=Inherit: Inherit via back propagation  FilterDenConstantOutMin=[]  FilterDenConstantOutMax=[]  PCopyOutDataTypeStr=Inherit: Inherit via back propagation  PCopyOutMin=[]  PCopyOutMax=[]  NCopyOutDataTypeStr=Inherit: Inherit via back propagation  NCopyOutMin=[]  NCopyOutMax=[]  IntegratorContinuousStateAttributes=''  IntegratorStateMustResolveToSignalObject=off  IntegratorRTWStateStorageClass=Auto  FilterContinuousStateAttributes=''  FilterStateMustResolveToSignalObject=off  FilterRTWStateStorageClass=Auto  ParallelPVariant=InternalParameters  IdealPVariant=Disabled  IVariant=Disabled  DVariant=Disabled  IntegratorVariant=Disabled  SatVariant=Disabled  AWVariant=Disabled  PCopyVariant=Disabled  TRVariant=Disabled  FdbkBlocksVariant=Forward  IdealPFdbkVariant=Disabled  SatFdbkVariant=Disabled  DerivativeFilterVariant=Disabled  NVariant=Disabled  NCopyVariant=Disabled_SignalSpec  FilterICVariant=Disabled  IntegratorICVariant=Disabled  ExternalResetVariant=Disabled  TRSumVariant=Passthrough  SumFdbkVariant=Disabled  SumVariant=Passthrough_P  TsampFilterVariant=InternalTs  TsampNgainVariant=Passthrough  TsampIntegralVariant=Disabled_SignalSpec  ExternalSaturationOutDataTypeStr=Inherit: Same as second input  DerivativeSourceVariant=Disabled  PreIntVariant=InternalPreInt
  PID Controller y : slpidlib/PID Controller  Controller=P  Form=Parallel  TimeDomain=Continuous-time  UseExternalTs=off  SampleTime=-1  IntegratorMethod=Forward Euler  FilterMethod=Forward Euler  ControllerParametersSource=internal  P=ctrl.Kpos(2,2)  I=ctrl.Kipos(2,2)  UseKiTs=off  D=0  UseExternalDerivativeSource=off  N=100  UseFilter=on  TunerSelectOption=Transfer Function Based (PID Tuner App)  InitialConditionSource=internal  InitialConditionForIntegrator=0  InitialConditionForFilter=0  DifferentiatorICPrevScaledInput=0  ExternalReset=none  TrackingMode=off  Kt=1  LimitOutput=off  SatLimitsSource=internal  UpperSaturationLimit=inf  LowerSaturationLimit=-inf  LinearizeAsGain=on  AntiWindupMode=none  Kb=1  LimitIntegrator=off  UpperIntegratorSaturationLimit=inf  LowerIntegratorSaturationLimit=-inf  POutMin=[]  POutMax=[]  IOutMin=[]  IOutMax=[]  DOutMin=[]  DOutMax=[]  NOutMin=[]  NOutMax=[]  SumOutMin=[]  SumOutMax=[]  SaturationOutMin=[]  SaturationOutMax=[]  PParamMin=[]  PParamMax=[]  IParamMin=[]  IParamMax=[]  DParamMin=[]  DParamMax=[]  NParamMin=[]  NParamMax=[]  KbParamMin=[]  KbParamMax=[]  KtParamMin=[]  KtParamMax=[]  KbOutMin=[]  KbOutMax=[]  KtOutMin=[]  KtOutMax=[]  IntegratorOutMin=[]  IntegratorOutMax=[]  FilterOutMin=[]  FilterOutMax=[]  SumI1OutMin=[]  SumI1OutMax=[]  SumI2OutMin=[]  SumI2OutMax=[]  SumI3OutMin=[]  SumI3OutMax=[]  SumI4OutMin=[]  SumI4OutMax=[]  SumDOutMin=[]  SumDOutMax=[]  DifferentiatorOutMin=[]  DifferentiatorOutMax=[]  FilterDiffOutCoefMin=[]  FilterDiffOutCoefMax=[]  ReciprocalOutMin=[]  ReciprocalOutMax=[]  SumDenOutMin=[]  SumDenOutMax=[]  SumNumOutMin=[]  SumNumOutMax=[]  DivideOutMin=[]  DivideOutMax=[]  UdiffTsProdOutMin=[]  UdiffTsProdOutMax=[]  NTsProdOutMin=[]  NTsProdOutMax=[]  UintegralTsProdOutMin=[]  UintegralTsProdOutMax=[]  UngainTsProdOutMin=[]  UngainTsProdOutMax=[]  ClampingZeroOutDataTypeStr=Inherit: Inherit via back propagation  ClampingZeroOutMin=[]  ClampingZeroOutMax=[]  FilterDenConstantOutDataTypeStr=Inherit: Inherit via back propagation  FilterDenConstantOutMin=[]  FilterDenConstantOutMax=[]  PCopyOutDataTypeStr=Inherit: Inherit via back propagation  PCopyOutMin=[]  PCopyOutMax=[]  NCopyOutDataTypeStr=Inherit: Inherit via back propagation  NCopyOutMin=[]  NCopyOutMax=[]  IntegratorContinuousStateAttributes=''  IntegratorStateMustResolveToSignalObject=off  IntegratorRTWStateStorageClass=Auto  FilterContinuousStateAttributes=''  FilterStateMustResolveToSignalObject=off  FilterRTWStateStorageClass=Auto  ParallelPVariant=InternalParameters  IdealPVariant=Disabled  IVariant=Disabled  DVariant=Disabled  IntegratorVariant=Disabled  SatVariant=Disabled  AWVariant=Disabled  PCopyVariant=Disabled  TRVariant=Disabled  FdbkBlocksVariant=Forward  IdealPFdbkVariant=Disabled  SatFdbkVariant=Disabled  DerivativeFilterVariant=Disabled  NVariant=Disabled  NCopyVariant=Disabled_SignalSpec  FilterICVariant=Disabled  IntegratorICVariant=Disabled  ExternalResetVariant=Disabled  TRSumVariant=Passthrough  SumFdbkVariant=Disabled  SumVariant=Passthrough_P  TsampFilterVariant=InternalTs  TsampNgainVariant=Passthrough  TsampIntegralVariant=Disabled_SignalSpec  ExternalSaturationOutDataTypeStr=Inherit: Same as second input  DerivativeSourceVariant=Disabled  PreIntVariant=InternalPreInt
  PID Controller z : slpidlib/PID Controller  Controller=P  Form=Parallel  TimeDomain=Continuous-time  UseExternalTs=off  SampleTime=-1  IntegratorMethod=Forward Euler  FilterMethod=Forward Euler  ControllerParametersSource=internal  P=ctrl.Kpos(3,3)  I=ctrl.Kipos(3,3)  UseKiTs=off  D=0  UseExternalDerivativeSource=off  N=100  UseFilter=on  TunerSelectOption=Transfer Function Based (PID Tuner App)  InitialConditionSource=internal  InitialConditionForIntegrator=0  InitialConditionForFilter=0  DifferentiatorICPrevScaledInput=0  ExternalReset=none  TrackingMode=off  Kt=1  LimitOutput=off  SatLimitsSource=internal  UpperSaturationLimit=inf  LowerSaturationLimit=-inf  LinearizeAsGain=on  AntiWindupMode=none  Kb=1  LimitIntegrator=off  UpperIntegratorSaturationLimit=inf  LowerIntegratorSaturationLimit=-inf  POutMin=[]  POutMax=[]  IOutMin=[]  IOutMax=[]  DOutMin=[]  DOutMax=[]  NOutMin=[]  NOutMax=[]  SumOutMin=[]  SumOutMax=[]  SaturationOutMin=[]  SaturationOutMax=[]  PParamMin=[]  PParamMax=[]  IParamMin=[]  IParamMax=[]  DParamMin=[]  DParamMax=[]  NParamMin=[]  NParamMax=[]  KbParamMin=[]  KbParamMax=[]  KtParamMin=[]  KtParamMax=[]  KbOutMin=[]  KbOutMax=[]  KtOutMin=[]  KtOutMax=[]  IntegratorOutMin=[]  IntegratorOutMax=[]  FilterOutMin=[]  FilterOutMax=[]  SumI1OutMin=[]  SumI1OutMax=[]  SumI2OutMin=[]  SumI2OutMax=[]  SumI3OutMin=[]  SumI3OutMax=[]  SumI4OutMin=[]  SumI4OutMax=[]  SumDOutMin=[]  SumDOutMax=[]  DifferentiatorOutMin=[]  DifferentiatorOutMax=[]  FilterDiffOutCoefMin=[]  FilterDiffOutCoefMax=[]  ReciprocalOutMin=[]  ReciprocalOutMax=[]  SumDenOutMin=[]  SumDenOutMax=[]  SumNumOutMin=[]  SumNumOutMax=[]  DivideOutMin=[]  DivideOutMax=[]  UdiffTsProdOutMin=[]  UdiffTsProdOutMax=[]  NTsProdOutMin=[]  NTsProdOutMax=[]  UintegralTsProdOutMin=[]  UintegralTsProdOutMax=[]  UngainTsProdOutMin=[]  UngainTsProdOutMax=[]  ClampingZeroOutDataTypeStr=Inherit: Inherit via back propagation  ClampingZeroOutMin=[]  ClampingZeroOutMax=[]  FilterDenConstantOutDataTypeStr=Inherit: Inherit via back propagation  FilterDenConstantOutMin=[]  FilterDenConstantOutMax=[]  PCopyOutDataTypeStr=Inherit: Inherit via back propagation  PCopyOutMin=[]  PCopyOutMax=[]  NCopyOutDataTypeStr=Inherit: Inherit via back propagation  NCopyOutMin=[]  NCopyOutMax=[]  IntegratorContinuousStateAttributes=''  IntegratorStateMustResolveToSignalObject=off  IntegratorRTWStateStorageClass=Auto  FilterContinuousStateAttributes=''  FilterStateMustResolveToSignalObject=off  FilterRTWStateStorageClass=Auto  ParallelPVariant=InternalParameters  IdealPVariant=Disabled  IVariant=Disabled  DVariant=Disabled  IntegratorVariant=Disabled  SatVariant=Disabled  AWVariant=Disabled  PCopyVariant=Disabled  TRVariant=Disabled  FdbkBlocksVariant=Forward  IdealPFdbkVariant=Disabled  SatFdbkVariant=Disabled  DerivativeFilterVariant=Disabled  NVariant=Disabled  NCopyVariant=Disabled_SignalSpec  FilterICVariant=Disabled  IntegratorICVariant=Disabled  ExternalResetVariant=Disabled  TRSumVariant=Passthrough  SumFdbkVariant=Disabled  SumVariant=Passthrough_P  TsampFilterVariant=InternalTs  TsampNgainVariant=Passthrough  TsampIntegralVariant=Disabled_SignalSpec  ExternalSaturationOutDataTypeStr=Inherit: Same as second input  DerivativeSourceVariant=Disabled  PreIntVariant=InternalPreInt
  Subsystem : Subsystem
  Terminator : Terminator
  v_c : Outport
  wires:
  PID Controller y/1 -> Mux/2
  Demux/2 -> PID Controller y/1
  e_p/1 -> Demux/1, Subsystem/1(e_p)
  Demux/3 -> PID Controller z/1
  PID Controller x/1 -> Mux/1
  PID Controller z/1 -> Mux/3
  Demux/1 -> PID Controller x/1
  Mux/1 -> v_c/1
  Constant/1 -> If/1
  If/1 -> Subsystem/Action
  If/2 -> Terminator/1

== system Simplified_UAV_Task3/Classic Position Controller/Sat ==
  In1 : Inport
  Demux : Demux  Outputs=3
  Mux : Mux  Inputs=3
  Saturation : Saturate  UpperLimit=12  LowerLimit=-12
  Saturation1 : Saturate  UpperLimit=12  LowerLimit=-12
  Saturation2 : Saturate  UpperLimit=12  LowerLimit=-12
  Scope : Scope
  Out1 : Outport
  wires:
  Mux/1 -> Scope/1, Out1/1
  In1/1 -> Demux/1
  Demux/3 -> Saturation/1
  Saturation/1 -> Mux/3
  Demux/2 -> Saturation2/1
  Demux/1 -> Saturation1/1
  Saturation1/1 -> Mux/1
  Saturation2/1 -> Mux/2
